simulink model "bincounter_3bit"  (R2022b)
settings: Solver=VariableStepAuto  StartTime=0.0  StopTime=inf  RelTol=1e-3
libraries: simulink_extras x4
settings Model: PacingRate=0.900000  Creator=F1  LastModifiedBy=Namratha
settings SolverCC: AlgebraicLoopSolver=TrustRegion
settings OptimizationCC: BooleanDataType=off
settings DebuggingCC: UnconnectedInputMsg=warning  UnconnectedOutputMsg=warning  UnconnectedLineMsg=warning  SFMachineParentedDataDiag=warning
settings ModelReferenceCC: EnableRefExpFcnMdlSchedulingChecks=on

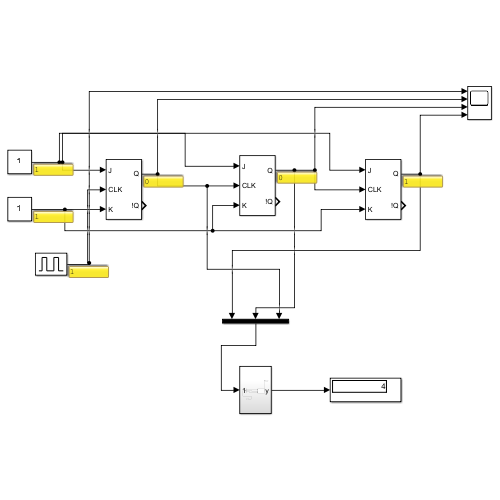
[thumbnail: Simulink's stored preview of the top-level diagram]
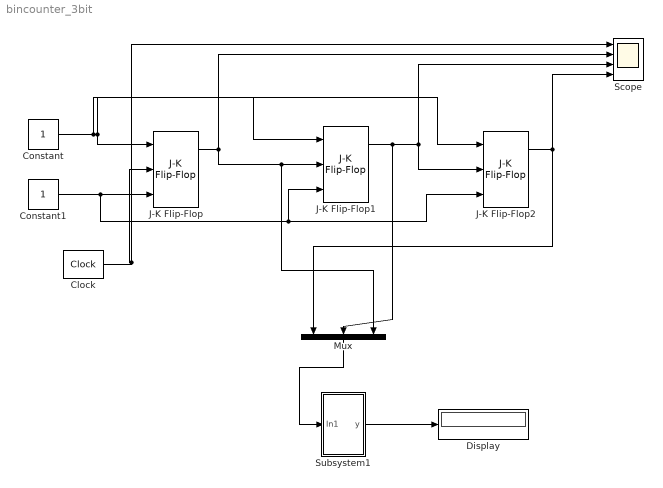
== system bincounter_3bit ==
  Clock : simulink_extras/Flip Flops/Clock  period=2
  Constant : Constant
  Constant1 : Constant
  Display : Display
  J-K Flip-Flop : simulink_extras/Flip Flops/J-K Flip-Flop  initial_condition=0
  J-K Flip-Flop1 : simulink_extras/Flip Flops/J-K Flip-Flop  initial_condition=0
  J-K Flip-Flop2 : simulink_extras/Flip Flops/J-K Flip-Flop  initial_condition=0
  Mux : Mux  Inputs=3
  Scope : Scope  NumInputPorts=4
  Subsystem1 : Subsystem
  wires:
  Constant/1 -> J-K Flip-Flop2/1, J-K Flip-Flop/1, J-K Flip-Flop1/1
  Constant1/1 -> J-K Flip-Flop2/3, J-K Flip-Flop1/3, J-K Flip-Flop/3
  Clock/1 -> J-K Flip-Flop/2, Scope/1
  J-K Flip-Flop/1 -> Scope/2, J-K Flip-Flop1/2, Mux/3
  J-K Flip-Flop1/1 -> J-K Flip-Flop2/2, Scope/3, Mux/2
  J-K Flip-Flop2/1 -> Scope/4, Mux/1
  Mux/1 -> Subsystem1/1(In1)
  Subsystem1/1(y) -> Display/1

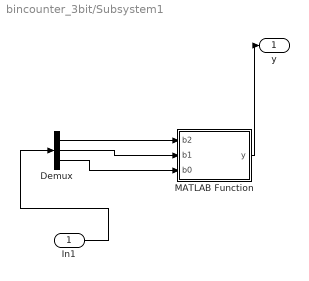
== system bincounter_3bit/Subsystem1 ==
  In1 : Inport
  Demux : Demux  Outputs=3
  MATLAB Function : MATLAB Function  TreatAsAtomicUnit=on
  y : Outport
  wires:
  Demux/2 -> MATLAB Function/2(b1)
  Demux/1 -> MATLAB Function/1(b2)
  Demux/3 -> MATLAB Function/3(b0)
  MATLAB Function/1(y) -> y/1
  In1/1 -> Demux/1

== matlab function bincounter_3bit/Subsystem1/MATLAB Function ==
  data: y output; b2 input; b1 input; b0 input
function y = fcn( b2   , b1    , b0    )
y =   b2*2^2 + b1*2^1 + b0*2^0 ;
end
